simulink model "netraSetuPipelineLive"  (R2026a)
settings: Solver=FixedStepDiscrete  StopTime=28800  FixedStep=5
model workspace (MAT data in the model file):
  CaptureSeconds = 90
  GradingConcurrency = 2
  GradingFailureRate = 0.05
  GradingSeconds = 39
  MaxAttempts = 3
  NumOphthalmologists = 2
  NumPhcs = 10
  QualityPassRate = 0.925925925926
  ReferableFraction = 0.3
  ReviewSecondsB = 30
  ReviewSecondsC = 240
  RngSeed = 42
  TierFractions = [0.384056903951 0.437547728282 0.178395367767]
  UploadSeconds = 29.6
settings Model: Creator=91740  LastModifiedBy=91740

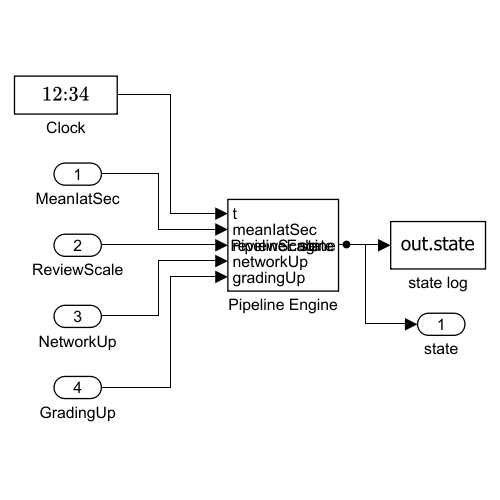
[thumbnail: Simulink's stored preview of the top-level diagram]
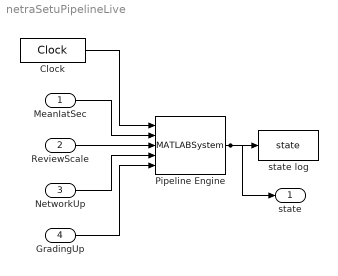
== system netraSetuPipelineLive ==
  MeanIatSec : Inport  OutDataTypeStr=double  PortDimensions=1  SampleTime=5
  ReviewScale : Inport  Port=2  OutDataTypeStr=double  PortDimensions=1  SampleTime=5
  NetworkUp : Inport  Port=3  OutDataTypeStr=double  PortDimensions=1  SampleTime=5
  GradingUp : Inport  Port=4  OutDataTypeStr=double  PortDimensions=1  SampleTime=5
  Clock : DigitalClock  SampleTime=5
  Pipeline Engine : MATLABSystem  System=PipelineEngine  NumPhcs=NumPhcs  NumOphthalmologists=NumOphthalmologists  GradingConcurrency=GradingConcurrency  CaptureSeconds=CaptureSeconds  QualityPassRate=QualityPassRate  UploadSeconds=UploadSeconds  GradingSeconds=GradingSeconds  GradingFailureRate=GradingFailureRate  MaxAttempts=MaxAttempts  TierFractions=TierFractions  ReviewSecondsB=ReviewSecondsB  ReviewSecondsC=ReviewSecondsC  ReferableFraction=ReferableFraction  RngSeed=RngSeed  MaxEntities=100000  MaxServers=50  MaxReviewers=8  CaptureQueueCapacity=200  SimulateUsing=Code generation
      mask Type: PipelineEngine
  state log : ToWorkspace  VariableName=state  SaveFormat=Timeseries  SampleTime=-1
  state : Outport
  wires:
  Clock/1 -> Pipeline Engine/1
  MeanIatSec/1 -> Pipeline Engine/2
  GradingUp/1 -> Pipeline Engine/5
  NetworkUp/1 -> Pipeline Engine/4
  ReviewScale/1 -> Pipeline Engine/3
  Pipeline Engine/1 -> state/1, state log/1
